simulink model "THREEPHAslx"  (R2021a)
settings: Solver=VariableStepAuto  StartTime=0.0  StopTime=10.0  RelTol=1e-3
undefined symbols (not defined in the file): powergui, spspowerguiLib
libraries: spsIGBTLib x6, simulink x3, spsMultimeterLib x3, spsThreePhaseVIMeasurementLib x3, spsThreePhaseParallelRLCBranchLib x2, spsDCVoltageSourceLib x1, spsGroundLib x1, spsSawtoothGeneratorLib x1, spsThreePhasePISectionLineLib x1, spsThreePhaseFaultLib x1, spsThreePhaseSourceLib x1
settings Model: Creator=shash  LastModifiedBy=Amit

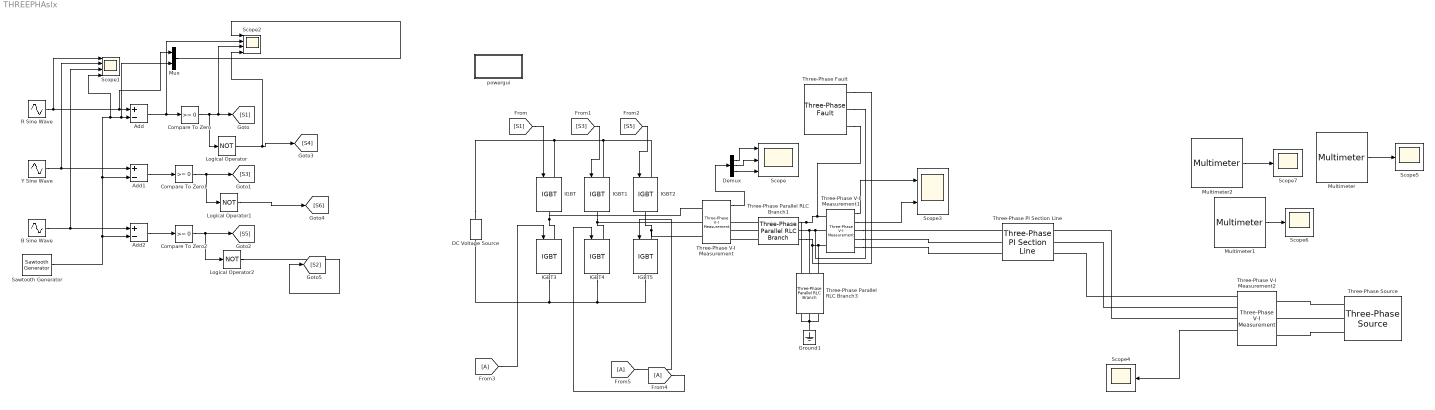
== system THREEPHAslx ==
  Add : Sum  Inputs=+-
  Add1 : Sum  Inputs=+-
  Add2 : Sum  Inputs=+-
  B Sine Wave : Sin  Frequency=2*pi*50  Phase=-2*pi/3  SampleTime=0
  Compare To Zero : simulink/Logic and Bit Operations/Compare To Zero  relop=>=  OutDataTypeStr=boolean
  Compare To Zero1 : simulink/Logic and Bit Operations/Compare To Zero  relop=>=  OutDataTypeStr=boolean
  Compare To Zero2 : simulink/Logic and Bit Operations/Compare To Zero  relop=>=  OutDataTypeStr=boolean
  DC Voltage Source : spsDCVoltageSourceLib/DC Voltage Source  Amplitude=100  Measurements=None
  Demux : Demux  Outputs=3
  Ground1 : spsGroundLib/Ground  LConnTagsString=a
  IGBT{,1..5} (6 alike) : spsIGBTLib/IGBT  Ron=0.001  Lon=0  Vf=1  Tf=1e-6  Tt=2e-6  IC=0  Rs=1e5  Cs=inf  Measurements=off
  Logical Operator : Logic  Operator=NOT  AllPortsSameDT=off  OutDataTypeStr=boolean
  Logical Operator1 : Logic  Operator=NOT  AllPortsSameDT=off  OutDataTypeStr=boolean
  Logical Operator2 : Logic  Operator=NOT  AllPortsSameDT=off  OutDataTypeStr=boolean
  Multimeter : spsMultimeterLib/Multimeter  PhasorSimulation=off  OutputType=Complex  sel=4  L=6  Gain=1  yselected={'Ib: Three-Phase Fault/Fault A'};  PSBOutputType=1  PSBequivalent=0  AxesSetting=[0,0.1,-100,100]  Display=0  SavedBlockNames=-11
  Multimeter1 : spsMultimeterLib/Multimeter  PhasorSimulation=off  OutputType=Complex  sel=5  L=6  Gain=1  yselected={'Ib: Three-Phase Fault/Fault B'};  PSBOutputType=1  PSBequivalent=0  AxesSetting=[0,0.1,-100,100]  Display=0  SavedBlockNames=-11
  Multimeter2 : spsMultimeterLib/Multimeter  PhasorSimulation=off  OutputType=Complex  sel=6  L=6  Gain=1  yselected={'Ib: Three-Phase Fault/Fault C'};  PSBOutputType=1  PSBequivalent=0  AxesSetting=[0,0.1,-100,100]  Display=0  SavedBlockNames=-11
  Mux : Mux  Inputs=2
  R Sine Wave : Sin  Frequency=2*pi*50  SampleTime=0
  Sawtooth Generator : spsSawtoothGeneratorLib/Sawtooth Generator  Freq=1e3  Phase=180  Ts=0
  Scope : Scope  NumInputPorts=3
  Scope1 : Scope  NumInputPorts=4
  Scope2 : Scope  NumInputPorts=4
  Scope3 : Scope  NumInputPorts=2
  Scope{4..7} (4 alike) : Scope
  Three-Phase PI Section Line : spsThreePhasePISectionLineLib/Three-Phase PI Section Line  LConnTagsString=a|b|c  RConnTagsString=A|B|C  Length=10  Frequency=50  Resistances=[ 0.01273 0.3864]  Inductances="[ 0.9337e-3  4.1264e-3]"  Capacitances=[12.74e-9 7.751e-9]
  Three-Phase Parallel RLC Branch1 : spsThreePhaseParallelRLCBranchLib/Three-Phase Parallel RLC Branch  LConnTagsString=A|B|C  RConnTagsString=A|B|C  BranchType=L  Resistance=1  Inductance=8.83e-3  Capacitance=1e-6  Measurements=None
      settings: SourceProductBaseCode=PS
  Three-Phase Parallel RLC Branch3 : spsThreePhaseParallelRLCBranchLib/Three-Phase Parallel RLC Branch  LConnTagsString=A|B|C  RConnTagsString=A|B|C  BranchType=C  Resistance=1  Inductance=.286e-3  Capacitance=2.86e-2  Measurements=None
      settings: SourceProductBaseCode=PS
  Three-Phase V-I Measurement : spsThreePhaseVIMeasurementLib/Three-Phase V-I Measurement  VoltageMeasurement=phase-to-ground  SetLabelV=off  LabelV=Vabc  Vpu=off  VpuLL=off  CurrentMeasurement=yes  SetLabelI=off  LabelI=Iabc  Ipu=off  Pbase=100e6  Vbase=500e3  OutputType=Complex  PhasorSimulation=off  PSBequivalent=0
  Three-Phase V-I Measurement1 : spsThreePhaseVIMeasurementLib/Three-Phase V-I Measurement  VoltageMeasurement=phase-to-ground  SetLabelV=off  LabelV=Vabc  Vpu=off  VpuLL=off  CurrentMeasurement=yes  SetLabelI=off  LabelI=Iabc  Ipu=off  Pbase=100e6  Vbase=500e3  OutputType=Complex  PhasorSimulation=off  PSBequivalent=0
  Three-Phase V-I Measurement2 : spsThreePhaseVIMeasurementLib/Three-Phase V-I Measurement  VoltageMeasurement=phase-to-ground  SetLabelV=off  LabelV=Vabc  Vpu=off  VpuLL=off  CurrentMeasurement=yes  SetLabelI=off  LabelI=Iabc  Ipu=off  Pbase=100e6  Vbase=500e3  OutputType=Complex  PhasorSimulation=off  PSBequivalent=0
  Three-Phase Fault : spsThreePhaseFaultLib/Three-Phase Fault  InitialStates=0  FaultA=on  FaultB=off  FaultC=off  GroundFault=on  SwitchTimes=[0.05 0.2]  External=off  SwitchStatus=NaN  FaultResistance=0.001  GroundResistance=0.01  SnubberResistance=1e6  SnubberCapacitance=inf  Measurements=Fault voltages and currents
  Three-Phase Source : spsThreePhaseSourceLib/Three-Phase Source  InternalConnection=Yg  VoltagePhases=off  Voltage=110  PhaseAngle=30  Voltage_phases=[25e3 25e3 25e3]/sqrt(3)  PhaseAngles_phases=[0 -120 +120]  Frequency=50  NonIdealSource=on  SpecifyImpedance=off  Resistance=0.8929  Inductance=16.58e-3  ShortCircuitLevel=100e6  BaseVoltage=25e3  XRratio=7  BusType=swing  Pref=10e3  Qref=0  Prefabc=[10e3, 10e3, 10e3]  Qrefabc=[0, 0, 0]  Qmin=-inf  Qmax=inf
  Y Sine Wave : Sin  Frequency=2*pi*50  Phase=2*pi/3  SampleTime=0
  powergui : Subsystem  Priority=1  AncestorBlock=spspowerguiLib/powergui  DialogController=POWERSYS.PowerSysDialog  InitFcn=powergui( 'InitFcn_Callback' , gcb , 0 , [ ] );  mask(PSB option menu block){SimulationMode=Continuous, SampleTime=50e-6, frequency=60, Iterations=50, frequencyindice=0, Pbase=100e6, ErrMax=1e-4, UnitsV=kV, UnitsW=MW, buscounter=0, FunctionMessages=off, echomessages=off, EnableUseOfTLC=off, CurrentSourceSwitches=off, DisableSnubberDevices=off, DisableRonSwitches=off, DisableVfSwitches=off, DisplayEquations=off, AutomaticDiscreteSolvers=off, SolverType=Tustin/Backward Euler (TBE), Interpol=off, ExternalGateDelay=off, methode=off, Ts=100, x0status=blocks, SPID=on, SwTol=0, HookPort=off, NonlinearTolerance=1e-4, nMaxIteration=100, ContinueOnMaxIteration=off, RestoreLinks=warning, ResistiveCurrentMeasurement=off, Frange=[0:2:500], Ylog=off, Xlog=on, ShowGrid=off, save=off, variable=ZData, structure=0, ZoomFFT=off, StartTime=0.0, cycles=1, DisplayStyle=1, fundamental=60, FreqAxis=off, MaxFrequency=1000, frequencyindicesteady=1, RmsSteady=1, display=off}
      mask prompts: SimulationMode "Simulation type:"; SampleTime "Sample time (s):"; frequency "Frequency (Hz):"; Iterations "Max iterations"; frequencyindice "Frequency (Hz)"; Pbase "Base power (VA)"; ErrMax "PQ tolerance (pu)"; UnitsV "Voltage units"; UnitsW "Power units"; buscounter "Load flow bus counter"; FunctionMessages "Disable Specialized Power Systems warnings"; echomessages "Display Specialized Power Systems compilation messages"; EnableUseOfTLC "Use TLC file when in Accelerator Simulation Mode and for code generation"; CurrentSourceSwitches "Disable ideal switching"; DisableSnubberDevices "Disable snubbers in switching devices"; DisableRonSwitches "Disable Ron resistances in switching devices"; DisableVfSwitches "Disable forward voltages in switching devices"; DisplayEquations "Display circuit differential equations"; AutomaticDiscreteSolvers "Automatically handle Discrete solver and Advanced tab solver settings of blocks"; SolverType "Discrete solver"; Interpol "Interpolate switching events"; ExternalGateDelay "Use time-stamped gate signals"; methode "Store switching topologies"; Ts "Buffer size (MBytes):"; x0status "Start simulation with initial electrical states from:"; SPID "Use ideal switching devices"; SwTol "Switch tolerance"; HookPort "Allow multiple powergui blocks"; NonlinearTolerance "Solver tolerance"; nMaxIteration "Maximum number of iterations"; ContinueOnMaxIteration "Continue Simulation if maximum number of iterations is reached"; RestoreLinks "Restore disabled links of Simscape Power Systems ST blocks:"; ResistiveCurrentMeasurement "Use non ideal current measurement blocks (1e-4Ohm internal resistance)"; Frange "Frequency Range"; Ylog "Log impedance"; Xlog "log Frequency"; ShowGrid "grid"; save "Save Data To Workspace"; variable "Variable Name"; structure "Structure Name (PSBFFTSCOPE)"; ZoomFFT "ZoomFFT (PSBFFTSCOPE)"; StartTime "Start Time (PSBFFTSCOPE)"; cycles "Cycles (PSBFFTSCOPE)"; DisplayStyle "Display style (PSBFFTSCOPE)"; fundamental "Fundamental (PSBFFTSCOPE)"; FreqAxis "Frequency Axis (PSBFFTSCOPE)"; MaxFrequency "Max Frequency (PSBFFTSCOPE)"; frequencyindicesteady "Frequency indice (STEADYSTATE)"; RmsSteady "RMS display (STEADYSTATE)"; display "Display Results"
      mask help: Set simulation type, simulation parameters, and preferences.
      mask init:
      | dispMessage = powergui('MaskInitialization',gcb,SimulationMode,SampleTime);
      settings: PreSaveFcn=powergui( 'PreSaveFcn_Callback' , gcb , [ ] , [ ] );  OpenFcn=sps_rtmsupport('OpenFcn',gcbh)
      mask Help: helpview(psbhelp)
      mask TypeOptions SimulationMode: Continuous | Discrete | Phasor | Discrete phasor
      mask Callback SimulationMode: powergui('SimulationType',[],[],gcb);
      mask TypeOptions UnitsV: V | kV
      mask TypeOptions UnitsW: W | kW | MW
      mask Callback CurrentSourceSwitches: powergui('SimulationType',[],[],gcb);
      mask Callback AutomaticDiscreteSolvers: powergui('SimulationType',[],[],gcb);
      mask TypeOptions SolverType: Tustin/Backward Euler (TBE) | Tustin | Backward Euler
      mask Callback SolverType: powergui('SimulationType',[],[],gcb);
      mask Callback Interpol: powergui('SimulationType',[],[],gcb);
      mask Callback ExternalGateDelay: powergui('SimulationType',[],[],gcb);
      mask Callback methode: powergui('SimulationType',[],[],gcb);
      mask TypeOptions x0status: blocks | steady | zero
      mask TypeOptions RestoreLinks: yes | warning | no
      mask Callback display: sps_rtmsupport('parametereditingmodes',gcbh) % Will be executed last in parameter callbacks to ensure mask enable consistency
      mask DialogControl SolverTab Prompt: Solver
      mask DialogControl AutoSolverNote Prompt: The Simulation type parameter is governed by Simulink. To access the Powergui solver settings, unselect auto (Automatic solver selection) solver in the Simulink solver options.
      mask DialogControl Container15 Prompt: Tools
      mask DialogControl StateAnalyzer Prompt: Measurements and States Analyzer
      mask DialogControl StateAnalyzer Callback: powerStates(bdroot(gcb))
      mask DialogControl RLCLineParameters Prompt: Power Line Parameters
      mask DialogControl RLCLineParameters Callback:
      | close_system(gcb)
      | powerLineParameters
      mask DialogControl DecouplingLines Prompt: Specify Decoupling Lines
      mask DialogControl DecouplingLines Tooltip: Click to replace selected Distributed Parameters Line blocks with Decoupling Line blocks
      mask DialogControl DecouplingLines Callback:
      | close_system(gcb);
      | DecouplingLineReplace(gcs)
      mask DialogControl LoadFlow Prompt: Load Flow Analyzer
      mask DialogControl LoadFlow Callback:
      | close_system(gcb)
      | powerLoadFlow
      mask DialogControl Container11 Prompt: Load Flow Parameters
      mask DialogControl MachineInitialization Prompt: Machine Initialization
      mask DialogControl MachineInitialization Callback:
      | close_system(gcb)
      | powericon('machineInitTool',bdroot(gcb),gcb)
      mask DialogControl ImpedanceMeasurement Prompt: Impedance Measurement
      mask DialogControl ImpedanceMeasurement Callback:
      | close_system(gcb)
      | power_zmeter(bdroot(gcb),gcb)
      mask DialogControl FFTAnalysis Prompt: FFT Analysis
      mask DialogControl FFTAnalysis Callback:
      | close_system(gcb)
      | power_fftscope(bdroot(gcb),gcb)
      mask DialogControl LinearSystemAnalyzer Prompt: Use Linear System Analyzer
      mask DialogControl LinearSystemAnalyzer Callback:
      | close_system(gcb)
      | power_ltiview(bdroot(gcb),gcb)
      mask DialogControl HysteresisDesign Prompt: Hysteresis Design
      mask DialogControl HysteresisDesign Callback:
      | close_system(gcb)
      | power_hysteresis(bdroot(gcb),gcb)
      mask DialogControl Control14 Prompt: Customize SPS blocks
      mask DialogControl Control14 Callback:
      | close_system(gcb);
      | power_customize;
      mask DialogControl GenerateReprot Prompt: Generate Report
      mask DialogControl GenerateReprot Callback:
      | close_system(gcb)
      | power_report(bdroot(gcb),gcb)
      mask DialogControl ParameterTabVar012 Prompt: Preferences
      mask DialogControl Solver Prompt: Solver
      mask DialogControl SolverDetails Prompt: Solver details for nonlinear elements
      mask Display: color('blue'),disp(dispMessage)
  wires:
  Three-Phase V-I Measurement1/1 -> Scope3/1
  Demux/1 -> Scope/1
  [S5] -> IGBT2/1
  [S1] -> IGBT/1
  [S3] -> IGBT1/1
  [A] -> IGBT5/1
  Three-Phase V-I Measurement/1 -> Demux/1
  Demux/2 -> Scope/2
  [A] -> IGBT3/1
  Demux/3 -> Scope/3
  [A] -> IGBT4/1
  Mux/1 -> Scope2/1
  Add2/1 -> Compare To Zero2/1
  Logical Operator1/1 -> [S6]
  Y Sine Wave/1 -> Scope1/2, Add1/1
  Compare To Zero1/1 -> Logical Operator1/1, [S3]
  Add1/1 -> Compare To Zero1/1
  Logical Operator2/1 -> [S2]
  R Sine Wave/1 -> Scope1/1, Mux/1, Add/1
  Compare To Zero/1 -> Logical Operator/1, Scope2/3, [S1]
  B Sine Wave/1 -> Scope1/3, Add2/1
  Sawtooth Generator/1 -> Add2/2, Add1/2, Scope1/4, Mux/2, Add/2
  Logical Operator/1 -> Scope2/4, [S4]
  Compare To Zero2/1 -> Logical Operator2/1, [S5]
  Add/1 -> Scope2/2, Compare To Zero/1
  Three-Phase V-I Measurement2/2 -> Scope4/1
  Multimeter1/1 -> Scope6/1
  Multimeter2/1 -> Scope7/1
  Multimeter/1 -> Scope5/1
  Three-Phase V-I Measurement1/2 -> Scope3/2
  connections:
  Three-Phase Parallel RLC Branch1/RConn3 -- Three-Phase Fault/LConn3 -- Three-Phase Parallel RLC Branch3/LConn3 -- Three-Phase V-I Measurement1/LConn3
  IGBT/RConn1 -- Three-Phase V-I Measurement/LConn1 -- IGBT3/LConn1
  IGBT4/RConn1 -- IGBT3/RConn1 -- DC Voltage Source/LConn1 -- IGBT5/RConn1
  IGBT5/LConn1 -- IGBT2/RConn1 -- Three-Phase V-I Measurement/LConn3
  Three-Phase V-I Measurement1/LConn2 -- Three-Phase Fault/LConn2 -- Three-Phase Parallel RLC Branch3/LConn2 -- Three-Phase Parallel RLC Branch1/RConn2
  Three-Phase Parallel RLC Branch3/RConn1 -- Three-Phase Parallel RLC Branch3/RConn3 -- Ground1/LConn1 -- Three-Phase Parallel RLC Branch3/RConn2
  DC Voltage Source/RConn1 -- IGBT/LConn1 -- IGBT2/LConn1 -- IGBT1/LConn1
  Three-Phase Parallel RLC Branch1/RConn1 -- Three-Phase Fault/LConn1 -- Three-Phase V-I Measurement1/LConn1 -- Three-Phase Parallel RLC Branch3/LConn1
  IGBT1/RConn1 -- Three-Phase V-I Measurement/LConn2 -- IGBT4/LConn1
  Three-Phase Parallel RLC Branch1/LConn2 -- Three-Phase V-I Measurement/RConn2
  Three-Phase Parallel RLC Branch1/LConn1 -- Three-Phase V-I Measurement/RConn1
  Three-Phase Parallel RLC Branch1/LConn3 -- Three-Phase V-I Measurement/RConn3
  Three-Phase V-I Measurement2/RConn1 -- Three-Phase PI Section Line/LConn1
  Three-Phase V-I Measurement2/RConn3 -- Three-Phase PI Section Line/LConn3
  Three-Phase Source/RConn2 -- Three-Phase V-I Measurement2/LConn2
  Three-Phase Source/RConn1 -- Three-Phase V-I Measurement2/LConn1
  Three-Phase V-I Measurement2/RConn2 -- Three-Phase PI Section Line/LConn2
  Three-Phase Source/RConn3 -- Three-Phase V-I Measurement2/LConn3
  Three-Phase V-I Measurement1/RConn1 -- Three-Phase PI Section Line/RConn1
  Three-Phase V-I Measurement1/RConn2 -- Three-Phase PI Section Line/RConn2
  Three-Phase V-I Measurement1/RConn3 -- Three-Phase PI Section Line/RConn3

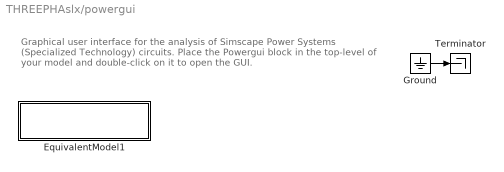
== system THREEPHAslx/powergui ==
  note: Graphical user interface for the analysis of
      | Simscape Power Systems (Specialized Technology) circuits.
      | Place the Powergui block in the top-level of your model and double-click
      | on it to open the GUI.
  EquivalentModel1 : Subsystem  mask{SwTol=SwTol}
      mask prompts: SwTol "SwitchTolerance"
      mask init:
      | S  = GetDataForEquivalentModel('SPID',gcbh,SwTol);
      mask Display:
      | color('blue')
      | disp('EQUIVALENT CIRCUIT\nSPID')
  Ground : Ground
  Terminator : Terminator
  wires:
  Ground/1 -> Terminator/1

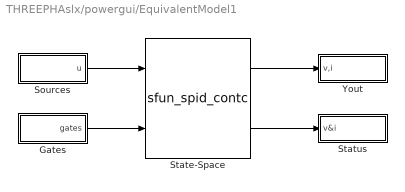
== system THREEPHAslx/powergui/EquivalentModel1 ==
  Gates : Subsystem
  Sources : Subsystem
  State-Space : S-Function  FunctionName=sfun_spid_contc  Parameters=S.Mg, [S.nb.x S.nb.u S.nb.y S.nb.s], S.x0, S.MgColNames, S.SwitchVf, S.SwitchType, S.SwitchGateInitialValue, S.SwitchTolerance,S.SaveMatrices,S.BufferSize  SFunctionDeploymentMode=off  EnableBusSupport=off
  Status : Subsystem
  Yout : Subsystem
  wires:
  State-Space/1 -> Yout/1(v,i)
  State-Space/2 -> Status/1(v&i)
  Gates/1(gates) -> State-Space/2
  Sources/1(u) -> State-Space/1

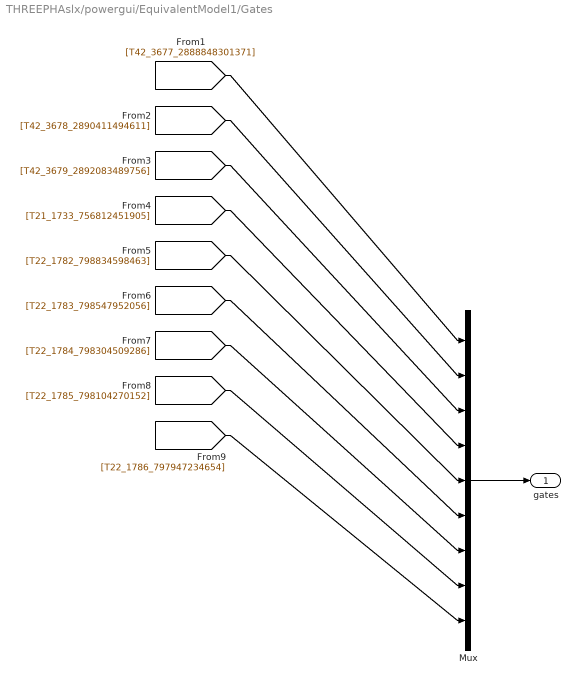
== system THREEPHAslx/powergui/EquivalentModel1/Gates ==
  Mux : Mux  Inputs=[1 1 1 1 1 1 1 1 1]
  gates : Outport  VectorParamsAs1DForOutWhenUnconnected=off
  wires:
  Mux/1 -> gates/1
  [T42_3677_2888848301371] -> Mux/1
  [T42_3678_2890411494611] -> Mux/2
  [T42_3679_2892083489756] -> Mux/3
  [T21_1733_756812451905] -> Mux/4
  [T22_1782_798834598463] -> Mux/5
  [T22_1783_798547952056] -> Mux/6
  [T22_1784_798304509286] -> Mux/7
  [T22_1785_798104270152] -> Mux/8
  [T22_1786_797947234654] -> Mux/9

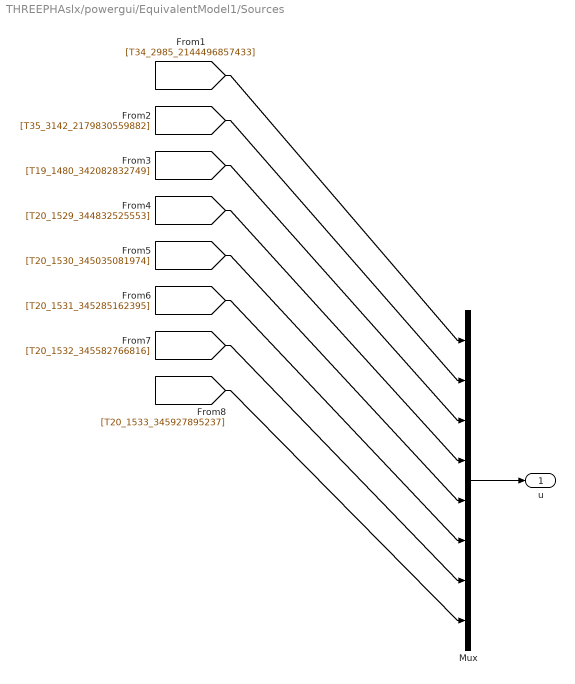
== system THREEPHAslx/powergui/EquivalentModel1/Sources ==
  Mux : Mux  Inputs=[1 3 1 1 1 1 1 1]
  u : Outport  VectorParamsAs1DForOutWhenUnconnected=off
  wires:
  Mux/1 -> u/1
  [T34_2985_2144496857433] -> Mux/1
  [T35_3142_2179830559882] -> Mux/2
  [T19_1480_342082832749] -> Mux/3
  [T20_1529_344832525553] -> Mux/4
  [T20_1530_345035081974] -> Mux/5
  [T20_1531_345285162395] -> Mux/6
  [T20_1532_345582766816] -> Mux/7
  [T20_1533_345927895237] -> Mux/8

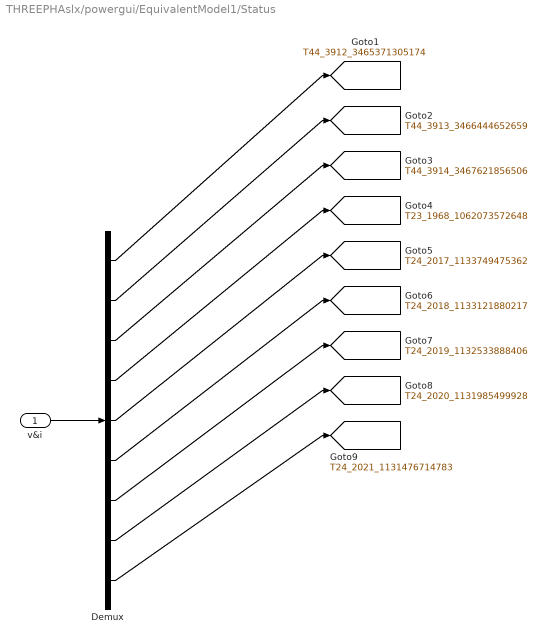
== system THREEPHAslx/powergui/EquivalentModel1/Status ==
  v&i : Inport
  Demux : Demux  Outputs=[2 2 2 2 2 2 2 2 2]
  tag scope: T23_1968_1062073572648=global, T24_2017_1133749475362=global, T24_2018_1133121880217=global, T24_2019_1132533888406=global, T24_2020_1131985499928=global, T24_2021_1131476714783=global, T44_3912_3465371305174=global, T44_3913_3466444652659=global, T44_3914_3467621856506=global
  wires:
  v&i/1 -> Demux/1
  Demux/1 -> [T44_3912_3465371305174]
  Demux/2 -> [T44_3913_3466444652659]
  Demux/3 -> [T44_3914_3467621856506]
  Demux/4 -> [T23_1968_1062073572648]
  Demux/5 -> [T24_2017_1133749475362]
  Demux/6 -> [T24_2018_1133121880217]
  Demux/7 -> [T24_2019_1132533888406]
  Demux/8 -> [T24_2020_1131985499928]
  Demux/9 -> [T24_2021_1131476714783]

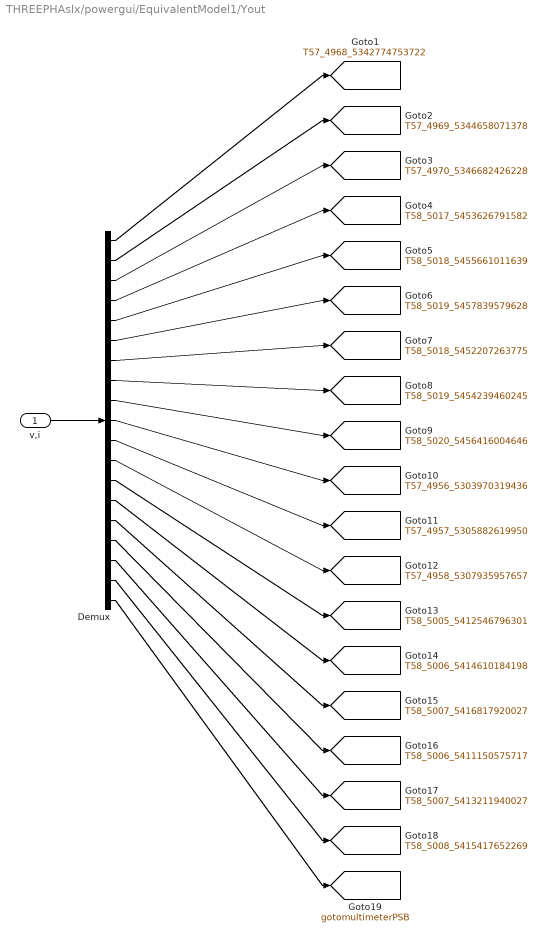
== system THREEPHAslx/powergui/EquivalentModel1/Yout ==
  v,i : Inport
  Demux : Demux  Outputs=[1 1 1 1 1 1 1 1 1 1 1 1 1 1 1 1 1 1 6]
  tag scope: T57_4956_5303970319436=global, T57_4957_5305882619950=global, T57_4958_5307935957657=global, T57_4968_5342774753722=global, T57_4969_5344658071378=global, T57_4970_5346682426228=global, T58_5005_5412546796301=global, T58_5006_5411150575717=global, T58_5006_5414610184198=global, T58_5007_5413211940027=global, T58_5007_5416817920027=global, T58_5008_5415417652269=global, T58_5017_5453626791582=global, T58_5018_5452207263775=global, T58_5018_5455661011639=global, T58_5019_5454239460245=global, T58_5019_5457839579628=global, T58_5020_5456416004646=global, gotomultimeterPSB=global
  wires:
  v,i/1 -> Demux/1
  Demux/1 -> [T57_4968_5342774753722]
  Demux/2 -> [T57_4969_5344658071378]
  Demux/3 -> [T57_4970_5346682426228]
  Demux/4 -> [T58_5017_5453626791582]
  Demux/5 -> [T58_5018_5455661011639]
  Demux/6 -> [T58_5019_5457839579628]
  Demux/7 -> [T58_5018_5452207263775]
  Demux/8 -> [T58_5019_5454239460245]
  Demux/9 -> [T58_5020_5456416004646]
  Demux/10 -> [T57_4956_5303970319436]
  Demux/11 -> [T57_4957_5305882619950]
  Demux/12 -> [T57_4958_5307935957657]
  Demux/13 -> [T58_5005_5412546796301]
  Demux/14 -> [T58_5006_5414610184198]
  Demux/15 -> [T58_5007_5416817920027]
  Demux/16 -> [T58_5006_5411150575717]
  Demux/17 -> [T58_5007_5413211940027]
  Demux/18 -> [T58_5008_5415417652269]
  Demux/19 -> [gotomultimeterPSB]
